simulink model "ComputedTorqueControl_20220607"  (R2020a)
settings: Solver=VariableStepAuto  StartTime=0.0  StopTime=12  FixedStep=0.01  RelTol=1e-3
undefined symbols (not defined in the file or in its folder): X, Y, Z
libraries: sm_lib x197, nesl_utility x84, sm_cable_robot_lib x44, simulink x1
(part 8 of 8)

== system ComputedTorqueControl_20220607/4-DOF CDPR/Frame2/Column 4/Lower Motor Assembly/Motor ==
  Double Bracket : Subsystem  AncestorBlock=sm_cable_robot_lib/Double Bracket  mask(Double Bracket){height=0.05, width=0.02, thickness=0.002, offset=0.13, holeOffset=0.04, holeRadius=0.005, rho=7800, color=[0.5 0.5 0.5]}
      mask prompts: height "Height (m)"; width "Width (m)"; thickness "Thickness (m)"; offset "Offset (m)"; holeOffset "Hole Offset (m)"; holeRadius "Hole Radius (m)"; rho "Density (kg/m^3)"; color "Color [r g b]"
      mask help:
      | This block models a double bracket element.
      |
      | Port B corresponds to the midpoint between the base faces of the two elements. Port H corresponds to the midpoint between the two holes.
      mask DialogControl Tab1 Prompt: Dimensions
      mask DialogControl Tab2 Prompt: Material Properties
      mask Display: image(fullfile(matlabroot,'toolbox','physmod','sm','smdemos','cable_robot','images','sm_cable_robot_double_bracket.png'));
  Flange : sm_lib/Body Elements/Cylindrical Solid  GraphicAmbientColor=[0.15 0.15 0.15 1.0]  BasedOnType=Density  CenterOfMass=[0 0 0]  CenterOfMassUnits=m  GraphicDiffuseColor=flangeColor  CylinderLength=flangeThickness  CylinderLengthUnits=m  CylinderRadius=flangeRadius  CylinderRadiusUnits=m  Density=housingRho  DensityUnits=kg/m^3  DoExposeReferenceFrame=off  GraphicEmissiveColor=[0.0 0.0 0.0 1.0]  ExportEntireGeometry=off  SerializedFrames=<Frames><Frame><Id>Frame1</Id><Value><Name>B</Name><Origin><Source>GeometricFeature</Source><FeatureName>bottom surface</FeatureName></Origin><PrimaryAxis><DefinedDirection>+Z</DefinedDirection><Source>ReferenceFrame</Source><SourceDirection>+Z</SourceDirection><FeatureName></FeatureName></PrimaryAxis><SecondaryAxis><DefinedDirection>+X</DefinedDirection><Source>ReferenceFrame</Source><SourceDirection>+X</SourceDirection><FeatureName></FeatureName></SecondaryAxis></Value></Frame></Frames>  MarkerShape=Sphere  MarkerSize=10  GraphicType=FromGeometry  InertiaType=CalculateFromGeometry  Mass=1  MassUnits=kg  MomentsOfInertia=[1 1 1]  MomentsOfInertiaUnits=kg*m^2  GraphicOpacity=1.0  ProductsOfInertia=[0 0 0]  ProductsOfInertiaUnits=kg*m^2  GraphicShininess=75  GraphicSpecularColor=[0.5 0.5 0.5 1.0]  GraphicVisPropType=SimpleVisualProperties
  Housing : sm_lib/Body Elements/Brick Solid  GraphicAmbientColor=[0.15 0.15 0.15 1.0]  BasedOnType=Density  BrickDimensions=[width height depth]  BrickDimensionUnits=m  CenterOfMass=[0 0 0]  CenterOfMassUnits=m  GraphicDiffuseColor=housingColor  Density=housingRho  DensityUnits=kg/m^3  DoExposeReferenceFrame=off  GraphicEmissiveColor=[0.0 0.0 0.0 1.0]  ExportEntireGeometry=off  SerializedFrames=<Frames><Frame><Id>Frame2</Id><Value><Name>B</Name><Origin><Source>GeometricFeature</Source><FeatureName>-y surface</FeatureName></Origin><PrimaryAxis><DefinedDirection>+Z</DefinedDirection><Source>ReferenceFrame</Source><SourceDirection>+Z</SourceDirection><FeatureName></FeatureName></PrimaryAxis><SecondaryAxis><DefinedDirection>+X</DefinedDirection><Source>ReferenceFrame</Source><SourceDirection>+X</SourceDirection><FeatureName></FeatureName></SecondaryAxis></Value></Frame><Frame><Id>Frame3</Id><Value><Name>F</Name><Origin><Source>GeometricFeature</Source><FeatureName>+z surface</FeatureName></Origin><PrimaryAxis><DefinedDirection>+Z</DefinedDirection><Source>ReferenceFrame</Source><SourceDirection>+Z</SourceDirection><FeatureName></FeatureName></PrimaryAxis><SecondaryAxis><DefinedDirection>+X</DefinedDirection><Source>ReferenceFrame</Source><SourceDirection>+X</SourceDirection><FeatureName></FeatureName></SecondaryAxis></Value></Frame></Frames>  MarkerShape=Sphere  MarkerSize=10  GraphicType=FromGeometry  InertiaType=CalculateFromGeometry  Mass=1  MassUnits=kg  MomentsOfInertia=[1 1 1]  MomentsOfInertiaUnits=kg*m^2  GraphicOpacity=1.0  ProductsOfInertia=[0 0 0]  ProductsOfInertiaUnits=kg*m^2  GraphicShininess=75  GraphicSpecularColor=[0.5 0.5 0.5 1.0]  GraphicVisPropType=SimpleVisualProperties
  Motor Revolute : sm_lib/Joints/Revolute Joint  JointMode=Normal  SenseConstraintForce=off  SenseConstraintForceX=off  SenseConstraintForceY=off  SenseConstraintForceZ=off  SenseConstraintTorque=off  SenseConstraintTorqueX=off  SenseConstraintTorqueY=off  SenseConstraintTorqueZ=off  SenseTotalForce=off  SenseTotalForceX=off  SenseTotalForceY=off  SenseTotalForceZ=off  SenseTotalTorque=off  SenseTotalTorqueX=off  SenseTotalTorqueY=off  SenseTotalTorqueZ=off  CompositeWrenchDir=FollowerOnBase  CompositeWrenchFrame=BaseFrame  EquilibriumPosition=0  EquilibriumPositionUnits=deg  SpringStiffness=0  SpringStiffnessUnits=N*m/deg  DampingCoefficient=0.01  DampingCoefficientUnits=N*m/(deg/s)  TorqueActuationMode=InputTorque  MotionActuationMode=ComputedMotion  SensePosition=on  SenseVelocity=on  SenseAcceleration=on  SenseTorqueForce=on  SenseLowerLimitTorqueForce=off  SenseUpperLimitTorqueForce=off  LowerLimitSpecify=off  LowerLimitBound=-90  LowerLimitBoundUnits=deg  LowerLimitStiffness=1e4  LowerLimitStiffnessUnits=N*m/deg  LowerLimitDamping=10  LowerLimitDampingUnits=N*m/(deg/s)  LowerLimitTransitionRegionWidth=0.1  LowerLimitTransitionRegionWidthUnits=deg  UpperLimitSpecify=off  UpperLimitBound=90  UpperLimitBoundUnits=deg  UpperLimitStiffness=1e4  UpperLimitStiffnessUnits=N*m/deg  UpperLimitDamping=10  UpperLimitDampingUnits=N*m/(deg/s)  UpperLimitTransitionRegionWidth=0.1  UpperLimitTransitionRegionWidthUnits=deg  PositionTargetSpecify=off  PositionTargetPriority=High  PositionTargetValue=0  PositionTargetValueUnits=deg  VelocityTargetSpecify=off  VelocityTargetPriority=High  VelocityTargetValue=0  VelocityTargetValueUnits=deg/s
  PS-Simulink Converter{1..4} (4 alike) : nesl_utility/PS-Simulink Converter  PhysicalDomain=network_engine_domain  SubClassName=ps_output  LeftPortType=input  RightPortType=output  PseudoPeriodic=off  Frequencies=[]  Unit=inherit  AffineConversion=off
  Rigid Transform : sm_lib/Frames and Transforms/Rigid Transform  TranslationMethod=Cartesian  TranslationStandardOffset=0  TranslationLengthUnit=m  TranslationStandardAxis=+Z  TranslationCartesianOffset=[0 -0.04 0.075]  TranslationROffset=0  TranslationROffsetUnits=m  TranslationZOffset=0  TranslationZOffsetUnits=m  TranslationThetaOffset=0  TranslationThetaOffsetUnits=deg  RotationMethod=RotationSequence  RotationAngleUnits=deg  RotationStandardAxis=+X  RotationAngle=90  RotationArbitraryAxis=[0 0 1]  FollAlignAxisA=+X  BaseAlignAxisA=+Y  FollAlignAxisB=+Y  BaseAlignAxisB=+Z  RotationSequenceAxes=FollowerAxes  RotationSequence=XYZ  RotationSequenceAngles=[-90 0 0]  RotationSequenceAnglesUnits=deg  RotationMatrix=[1 0 0; 0 1 0; 0 0 1]
  Shaft : sm_lib/Body Elements/Cylindrical Solid  GraphicAmbientColor=[0.15 0.15 0.15 1.0]  BasedOnType=Density  CenterOfMass=[0 0 0.075]  CenterOfMassUnits=m  GraphicDiffuseColor=shaftColor  CylinderLength=shaftLength  CylinderLengthUnits=m  CylinderRadius=shaftRadius  CylinderRadiusUnits=m  Density=shaftRho  DensityUnits=kg/m^3  DoExposeReferenceFrame=on  GraphicEmissiveColor=[0.0 0.0 0.0 1.0]  ExportEntireGeometry=off  SerializedFrames=<Frames><Frame><Id>Frame1</Id><Value><Name>B</Name><Origin><Source>GeometricFeature</Source><FeatureName>bottom surface</FeatureName></Origin><PrimaryAxis><DefinedDirection>+Z</DefinedDirection><Source>ReferenceFrame</Source><SourceDirection>+Z</SourceDirection><FeatureName></FeatureName></PrimaryAxis><SecondaryAxis><DefinedDirection>+X</DefinedDirection><Source>ReferenceFrame</Source><SourceDirection>+X</SourceDirection><FeatureName></FeatureName></SecondaryAxis></Value></Frame></Frames>  MarkerShape=Sphere  MarkerSize=10  GraphicType=FromGeometry  InertiaType=Custom  Mass=0.09189  MassUnits=kg  MomentsOfInertia=[0 0 1.149e-6]  MomentsOfInertiaUnits=kg*m^2  GraphicOpacity=1.0  ProductsOfInertia=[0 0 0]  ProductsOfInertiaUnits=kg*m^2  GraphicShininess=75  GraphicSpecularColor=[0.5 0.5 0.5 1.0]  GraphicVisPropType=SimpleVisualProperties
  Simulink-PS Converter : nesl_utility/Simulink-PS Converter  PhysicalDomain=network_engine_domain  SubClassName=ps_input  LeftPortType=input  RightPortType=output  PseudoPeriodic=off  Frequencies=[]  NoiseDistribution=none  NoiseParameters=[]  Unit=N*m  AffineConversion=off  FilteringAndDerivatives=filter  SimscapeFilterOrder=2  InputFilterTimeConstant=0.001  UdotUserProvided=0
  To Workspace1 : ToWorkspace  VariableName=qD  SaveFormat=Structure With Time  SampleTime=-1
  To Workspace2 : ToWorkspace  VariableName=dqD  SaveFormat=Structure With Time  SampleTime=-1
  To Workspace3 : ToWorkspace  VariableName=ddqD  SaveFormat=Structure With Time  SampleTime=-1
  To Workspace4 : ToWorkspace  VariableName=Dtrq  SaveFormat=Structure With Time  SampleTime=-1
  B : PMIOPort  Side=Left
  S : PMIOPort  Port=2  Side=Right
  tag scope: Dtrq=global, ddqD=global, dqD=global, qD=global
  wires:
  [DInTorque] -> Simulink-PS Converter/1
  PS-Simulink Converter3/1 -> To Workspace3/1, [ddqD]
  PS-Simulink Converter2/1 -> To Workspace2/1, [dqD]
  PS-Simulink Converter4/1 -> To Workspace4/1, [Dtrq]
  PS-Simulink Converter1/1 -> To Workspace1/1, [qD]
  connections:
  Housing/LConn1 -- B/RConn1
  S/RConn1 -- Shaft/RConn1
  Shaft/LConn1 -- Motor Revolute/RConn1
  Flange/LConn1 -- Housing/RConn1 -- Rigid Transform/LConn1 -- Motor Revolute/LConn1
  Rigid Transform/RConn1 -- Double Bracket/LConn1
  Simulink-PS Converter/RConn1 -- Motor Revolute/LConn2
  PS-Simulink Converter3/LConn1 -- Motor Revolute/RConn4
  PS-Simulink Converter1/LConn1 -- Motor Revolute/RConn2
  PS-Simulink Converter4/LConn1 -- Motor Revolute/RConn5
  PS-Simulink Converter2/LConn1 -- Motor Revolute/RConn3

== system ComputedTorqueControl_20220607/4-DOF CDPR/Frame2/Column 4/Lower Motor Assembly/Pulley and Bracket Assembly ==
  Pulley : sm_cable_robot_lib/Pulley  radius=0.02  thickness=0.12  holeRadius=0.005  grooveDepth=0.004  grooveWidth=0.1  grooveAngle=25  rho=7800  color=[0.7 0.7 0.7]  markerColor=[0.3 0.3 0.3]
      link override Pulley: CenterOfMass=[0 0 0.1]  InertiaType=Custom  Mass=1.8378  MomentsOfInertia=[0 0 3.905e-4]
      settings: SourceProductBaseCode=MS
  Rigid Transform1 : sm_lib/Frames and Transforms/Rigid Transform  TranslationMethod=None  TranslationStandardOffset=0  TranslationLengthUnit=m  TranslationStandardAxis=+Z  TranslationCartesianOffset=[0 0 0]  TranslationROffset=0  TranslationROffsetUnits=m  TranslationZOffset=0  TranslationZOffsetUnits=m  TranslationThetaOffset=0  TranslationThetaOffsetUnits=deg  RotationMethod=None  RotationAngleUnits=deg  RotationStandardAxis=+X  RotationAngle=90  RotationArbitraryAxis=[0 0 1]  FollAlignAxisA=+X  BaseAlignAxisA=+Y  FollAlignAxisB=+Y  BaseAlignAxisB=+Z  RotationSequenceAxes=FollowerAxes  RotationSequence=XYZ  RotationSequenceAngles=[-90 0 0]  RotationSequenceAnglesUnits=deg  RotationMatrix=[1 0 0; 0 1 0; 0 0 1]
  B : PMIOPort  Side=Left
  connections:
  Rigid Transform1/RConn1 -- Pulley/LConn1
  B/RConn1 -- Rigid Transform1/LConn1

== system ComputedTorqueControl_20220607/4-DOF CDPR/Frame2/Column 1/Lower Motor Assembly/Motor/Double Bracket ==
  Base Center Frame : sm_lib/Frames and Transforms/Reference Frame
  Left Bracket : sm_cable_robot_lib/Bracket  height=height  width=width  thickness=thickness  holeOffset=holeOffset  holeRadius=holeRadius  rho=rho  color=color
      settings: SourceProductBaseCode=MS
  Left Bracket xForm : sm_lib/Frames and Transforms/Rigid Transform  TranslationMethod=StandardAxis  TranslationStandardOffset=0.5*offset  TranslationLengthUnit=m  TranslationStandardAxis=-Y  TranslationCartesianOffset=[0 0 0]  TranslationROffset=0  TranslationROffsetUnits=m  TranslationZOffset=0  TranslationZOffsetUnits=m  TranslationThetaOffset=0  TranslationThetaOffsetUnits=deg  RotationMethod=AlignedAxes  RotationAngleUnits=deg  RotationStandardAxis=+X  RotationAngle=90  RotationArbitraryAxis=[0 0 1]  FollAlignAxisA=+X  BaseAlignAxisA=+X  FollAlignAxisB=+Y  BaseAlignAxisB=+Z  RotationSequenceAxes=FollowerAxes  RotationSequence=XYX  RotationSequenceAngles=[0 0 0]  RotationSequenceAnglesUnits=deg  RotationMatrix=[1 0 0; 0 1 0; 0 0 1]
  Right Bracket : sm_cable_robot_lib/Bracket  height=height  width=width  thickness=thickness  holeOffset=holeOffset  holeRadius=holeRadius  rho=rho  color=color
      settings: SourceProductBaseCode=MS
  Right Bracket xForm : sm_lib/Frames and Transforms/Rigid Transform  TranslationMethod=StandardAxis  TranslationStandardOffset=0.5*offset  TranslationLengthUnit=m  TranslationStandardAxis=+Y  TranslationCartesianOffset=[0 0 0]  TranslationROffset=0  TranslationROffsetUnits=m  TranslationZOffset=0  TranslationZOffsetUnits=m  TranslationThetaOffset=0  TranslationThetaOffsetUnits=deg  RotationMethod=AlignedAxes  RotationAngleUnits=deg  RotationStandardAxis=+X  RotationAngle=90  RotationArbitraryAxis=[0 0 1]  FollAlignAxisA=+X  BaseAlignAxisA=+X  FollAlignAxisB=+Y  BaseAlignAxisB=+Z  RotationSequenceAxes=FollowerAxes  RotationSequence=XYX  RotationSequenceAngles=[0 0 0]  RotationSequenceAnglesUnits=deg  RotationMatrix=[1 0 0; 0 1 0; 0 0 1]
  B : PMIOPort  Side=Left
  connections:
  B/RConn1 -- Base Center Frame/RConn1 -- Right Bracket xForm/LConn1 -- Left Bracket xForm/LConn1
  Right Bracket/LConn1 -- Right Bracket xForm/RConn1
  Left Bracket/LConn1 -- Left Bracket xForm/RConn1

== system ComputedTorqueControl_20220607/4-DOF CDPR/Frame2/Column 2/Lower Motor Assembly1/Motor/Double Bracket ==
  Base Center Frame : sm_lib/Frames and Transforms/Reference Frame
  Left Bracket : sm_cable_robot_lib/Bracket  height=height  width=width  thickness=thickness  holeOffset=holeOffset  holeRadius=holeRadius  rho=rho  color=color
      settings: SourceProductBaseCode=MS
  Left Bracket xForm : sm_lib/Frames and Transforms/Rigid Transform  TranslationMethod=StandardAxis  TranslationStandardOffset=0.5*offset  TranslationLengthUnit=m  TranslationStandardAxis=-Y  TranslationCartesianOffset=[0 0 0]  TranslationROffset=0  TranslationROffsetUnits=m  TranslationZOffset=0  TranslationZOffsetUnits=m  TranslationThetaOffset=0  TranslationThetaOffsetUnits=deg  RotationMethod=AlignedAxes  RotationAngleUnits=deg  RotationStandardAxis=+X  RotationAngle=90  RotationArbitraryAxis=[0 0 1]  FollAlignAxisA=+X  BaseAlignAxisA=+X  FollAlignAxisB=+Y  BaseAlignAxisB=+Z  RotationSequenceAxes=FollowerAxes  RotationSequence=XYX  RotationSequenceAngles=[0 0 0]  RotationSequenceAnglesUnits=deg  RotationMatrix=[1 0 0; 0 1 0; 0 0 1]
  Right Bracket : sm_cable_robot_lib/Bracket  height=height  width=width  thickness=thickness  holeOffset=holeOffset  holeRadius=holeRadius  rho=rho  color=color
      settings: SourceProductBaseCode=MS
  Right Bracket xForm : sm_lib/Frames and Transforms/Rigid Transform  TranslationMethod=StandardAxis  TranslationStandardOffset=0.5*offset  TranslationLengthUnit=m  TranslationStandardAxis=+Y  TranslationCartesianOffset=[0 0 0]  TranslationROffset=0  TranslationROffsetUnits=m  TranslationZOffset=0  TranslationZOffsetUnits=m  TranslationThetaOffset=0  TranslationThetaOffsetUnits=deg  RotationMethod=AlignedAxes  RotationAngleUnits=deg  RotationStandardAxis=+X  RotationAngle=90  RotationArbitraryAxis=[0 0 1]  FollAlignAxisA=+X  BaseAlignAxisA=+X  FollAlignAxisB=+Y  BaseAlignAxisB=+Z  RotationSequenceAxes=FollowerAxes  RotationSequence=XYX  RotationSequenceAngles=[0 0 0]  RotationSequenceAnglesUnits=deg  RotationMatrix=[1 0 0; 0 1 0; 0 0 1]
  B : PMIOPort  Side=Left
  connections:
  B/RConn1 -- Base Center Frame/RConn1 -- Right Bracket xForm/LConn1 -- Left Bracket xForm/LConn1
  Right Bracket/LConn1 -- Right Bracket xForm/RConn1
  Left Bracket/LConn1 -- Left Bracket xForm/RConn1

== system ComputedTorqueControl_20220607/4-DOF CDPR/Frame2/Column 3/Lower Motor Assembly/Motor/Double Bracket ==
  Base Center Frame : sm_lib/Frames and Transforms/Reference Frame
  Left Bracket : sm_cable_robot_lib/Bracket  height=height  width=width  thickness=thickness  holeOffset=holeOffset  holeRadius=holeRadius  rho=rho  color=color
      settings: SourceProductBaseCode=MS
  Left Bracket xForm : sm_lib/Frames and Transforms/Rigid Transform  TranslationMethod=StandardAxis  TranslationStandardOffset=0.5*offset  TranslationLengthUnit=m  TranslationStandardAxis=-Y  TranslationCartesianOffset=[0 0 0]  TranslationROffset=0  TranslationROffsetUnits=m  TranslationZOffset=0  TranslationZOffsetUnits=m  TranslationThetaOffset=0  TranslationThetaOffsetUnits=deg  RotationMethod=AlignedAxes  RotationAngleUnits=deg  RotationStandardAxis=+X  RotationAngle=90  RotationArbitraryAxis=[0 0 1]  FollAlignAxisA=+X  BaseAlignAxisA=+X  FollAlignAxisB=+Y  BaseAlignAxisB=+Z  RotationSequenceAxes=FollowerAxes  RotationSequence=XYX  RotationSequenceAngles=[0 0 0]  RotationSequenceAnglesUnits=deg  RotationMatrix=[1 0 0; 0 1 0; 0 0 1]
  Right Bracket : sm_cable_robot_lib/Bracket  height=height  width=width  thickness=thickness  holeOffset=holeOffset  holeRadius=holeRadius  rho=rho  color=color
      settings: SourceProductBaseCode=MS
  Right Bracket xForm : sm_lib/Frames and Transforms/Rigid Transform  TranslationMethod=StandardAxis  TranslationStandardOffset=0.5*offset  TranslationLengthUnit=m  TranslationStandardAxis=+Y  TranslationCartesianOffset=[0 0 0]  TranslationROffset=0  TranslationROffsetUnits=m  TranslationZOffset=0  TranslationZOffsetUnits=m  TranslationThetaOffset=0  TranslationThetaOffsetUnits=deg  RotationMethod=AlignedAxes  RotationAngleUnits=deg  RotationStandardAxis=+X  RotationAngle=90  RotationArbitraryAxis=[0 0 1]  FollAlignAxisA=+X  BaseAlignAxisA=+X  FollAlignAxisB=+Y  BaseAlignAxisB=+Z  RotationSequenceAxes=FollowerAxes  RotationSequence=XYX  RotationSequenceAngles=[0 0 0]  RotationSequenceAnglesUnits=deg  RotationMatrix=[1 0 0; 0 1 0; 0 0 1]
  B : PMIOPort  Side=Left
  connections:
  B/RConn1 -- Base Center Frame/RConn1 -- Right Bracket xForm/LConn1 -- Left Bracket xForm/LConn1
  Right Bracket/LConn1 -- Right Bracket xForm/RConn1
  Left Bracket/LConn1 -- Left Bracket xForm/RConn1

== system ComputedTorqueControl_20220607/4-DOF CDPR/Frame2/Column 4/Lower Motor Assembly/Motor/Double Bracket ==
  Base Center Frame : sm_lib/Frames and Transforms/Reference Frame
  Left Bracket : sm_cable_robot_lib/Bracket  height=height  width=width  thickness=thickness  holeOffset=holeOffset  holeRadius=holeRadius  rho=rho  color=color
      settings: SourceProductBaseCode=MS
  Left Bracket xForm : sm_lib/Frames and Transforms/Rigid Transform  TranslationMethod=StandardAxis  TranslationStandardOffset=0.5*offset  TranslationLengthUnit=m  TranslationStandardAxis=-Y  TranslationCartesianOffset=[0 0 0]  TranslationROffset=0  TranslationROffsetUnits=m  TranslationZOffset=0  TranslationZOffsetUnits=m  TranslationThetaOffset=0  TranslationThetaOffsetUnits=deg  RotationMethod=AlignedAxes  RotationAngleUnits=deg  RotationStandardAxis=+X  RotationAngle=90  RotationArbitraryAxis=[0 0 1]  FollAlignAxisA=+X  BaseAlignAxisA=+X  FollAlignAxisB=+Y  BaseAlignAxisB=+Z  RotationSequenceAxes=FollowerAxes  RotationSequence=XYX  RotationSequenceAngles=[0 0 0]  RotationSequenceAnglesUnits=deg  RotationMatrix=[1 0 0; 0 1 0; 0 0 1]
  Right Bracket : sm_cable_robot_lib/Bracket  height=height  width=width  thickness=thickness  holeOffset=holeOffset  holeRadius=holeRadius  rho=rho  color=color
      settings: SourceProductBaseCode=MS
  Right Bracket xForm : sm_lib/Frames and Transforms/Rigid Transform  TranslationMethod=StandardAxis  TranslationStandardOffset=0.5*offset  TranslationLengthUnit=m  TranslationStandardAxis=+Y  TranslationCartesianOffset=[0 0 0]  TranslationROffset=0  TranslationROffsetUnits=m  TranslationZOffset=0  TranslationZOffsetUnits=m  TranslationThetaOffset=0  TranslationThetaOffsetUnits=deg  RotationMethod=AlignedAxes  RotationAngleUnits=deg  RotationStandardAxis=+X  RotationAngle=90  RotationArbitraryAxis=[0 0 1]  FollAlignAxisA=+X  BaseAlignAxisA=+X  FollAlignAxisB=+Y  BaseAlignAxisB=+Z  RotationSequenceAxes=FollowerAxes  RotationSequence=XYX  RotationSequenceAngles=[0 0 0]  RotationSequenceAnglesUnits=deg  RotationMatrix=[1 0 0; 0 1 0; 0 0 1]
  B : PMIOPort  Side=Left
  connections:
  B/RConn1 -- Base Center Frame/RConn1 -- Right Bracket xForm/LConn1 -- Left Bracket xForm/LConn1
  Right Bracket/LConn1 -- Right Bracket xForm/RConn1
  Left Bracket/LConn1 -- Left Bracket xForm/RConn1

== matlab function ComputedTorqueControl_20220607/Reference Trajectory Generator/Subsystem/MATLAB Function2 ==
  data: t input; Adq output; Bdq output; Cdq output; Ddq output
function [Adq,Bdq,Cdq,Ddq] = fcn(t)

 Adq=(-t+2).*(0<=t&&t<=4)+(t-8).*(4<=t&&t<=12);
 Bdq=(-t+4).*(0<=t&&t<=8)+(t-10).*(8<=t&&t<=12);
 Cdq=(t-2).*(0<=t&&t<=4)+(-t+8).*(4<=t&&t<=12);
 Ddq=(t-4).*(0<=t&&t<=8)+(-t+10).*(8<=t&&t<=12);
end

== matlab function ComputedTorqueControl_20220607/Reference Trajectory Generator/Subsystem/MATLAB Function1 ==
  data: t input; Aq output; Bq output; Cq output; Dq output
function [Aq,Bq,Cq,Dq] = fcn(t)

  Aq=(-0.5*(t-2)^2+2).*(0<=t&&t<4)+(0.5*(t-8)^2-8).*(4<=t&&t<12);
  Bq=(-0.5*(t-4)^2+8).*(0<=t&&t<8)+(0.5*(t-10)^2-2).*(8<t&&t<12);
  Cq=(0.5*(t-2)^2-2).*(0<t&&t<=4)+(-0.5*(t-8)^2+8).* (4<t&&t<12);
  Dq=(0.5*(t-4)^2-8).*(0<t&&t<=8)+(-0.5*(t-10)^2+2).* (8<t&&t<12);
 
end

== matlab function ComputedTorqueControl_20220607/Reference Trajectory Generator/Subsystem/MATLAB Function3 ==
  data: t input; Addq output; Bddq output; Cddq output; Dddq output
function [Addq,Bddq,Cddq,Dddq] = fcn(t)

Addq=-1.801*t+11.63;
Bddq=-4.122*t+38.26;
Cddq=1.801*t-11.63;
Dddq=4.122*t-38.26;

end

== matlab function ComputedTorqueControl_20220607/Reference Trajectory Generator/Subsystem/MATLAB Function4 ==
  data: t input; Aq output; Bq output; Cq output; Dq output
function [Aq,Bq,Cq,Dq] = fcn(t)

  Aq=3.994*sin(0.1796*t-2.995) + 4.244*sin(0.5746*t+0.1555);
  Bq=19.81*sin(0.002025*t+2.993) + 5.099*sin(0.5257*t-0.6065);
  Cq=18.34*sin(0.002452*t+0.1331) + 5.084*sin(0.5268*t-2.588);
  Dq=4.038*sin(0.1823*t+0.1823) + 4.202*sin(0.5769*t+2.34);
 
end

== matlab function ComputedTorqueControl_20220607/Reference Trajectory Generator/Subsystem/MATLAB Function ==
  data: t input; Atau output; Btau output; Ctau output; Dtau output
function [Atau,Btau,Ctau,Dtau] = fcn(t)

Atau= 2.721*sin(0.525*t+2.124);
Btau=2.724*sin(0.5233*t+0.9912);
Ctau=2.727*sin(0.5209*t-0.9968);
Dtau=2.722*sin(0.5277*t-2.18);

end

== matlab function ComputedTorqueControl_20220607/Tension Force ==
  data: q input; f output; al input; be input; ga input
function f = Tension_Force(q,al,be,ga)

% %定义的电机转角q;q=[q1;q2;q3;q4];
q1=q(1);q2=q(2);q3=q(3);q4=q(4);

 % %定义的零位置的悬索（未形变）长度L00：
L0=[2.0992    1.9280    1.5225    1.6912    2.0992    1.9280    1.5225    1.6912]';
l01=L0(1,1);l02=L0(2,1);l03=L0(3,1);l04=L0(4,1);
l05=L0(5,1);l06=L0(6,1);l07=L0(7,1);l08=L0(8,1);
 
% %⑥悬索未形变的长度Lo。初始点位置为[0；0；1.1；0；0；0]。
% l0=1.7305*a0;
r0=0.02;
% m0=5.826*10^(-4);
lo1=l01+r0*q1;lo2=l02+r0*q2;lo3=l03+r0*q3;lo4=l04+r0*q4;
lo5=l05+r0*q1;lo6=l06+r0*q2;lo7=l07+r0*q3;lo8=l08+r0*q4;

%执行器位置参数
x=1.1;y=1.5;z=0.75;
%外框架尺寸设定
A=2.2;B=3.0;C=1.5;
a=0.2;b=0.05;h=0.1;


P=[x;y;z];
% R=[cos(ga),-sin(ga),0;sin(ga),cos(ga),0;0,0,1];
R=[cos(ga)*cos(be),  cos(ga)*sin(be)*sin(al)-sin(ga)*cos(al),  cos(ga)*sin(be)*cos(al)+sin(ga)*sin(al);  
   sin(ga)*cos(be),  sin(ga)*sin(be)*sin(al)+cos(ga)*cos(al),  sin(ga)*sin(be)*cos(al)-cos(ga)*sin(al);   
          -sin(be),                          cos(be)*sin(al),                        cos(be)*cos(al)   ];       
% %全局坐标原点O位于外框架接地平面中心。局部坐标系原点建立在末端执行器中心。
B1=[A/2;B/2;   C];B2=[-A/2;B/2;   C];B3=[-A/2;-B/2;   C];B4=[A/2;-B/2;  C];
B5=[A/2;B/2; C-h];B6=[-A/2;B/2; C-h];B7=[-A/2;-B/2; C-h];B8=[A/2;-B/2; C-h];
p1=[a/2;b/2; h/2];p2=[-a/2;b/2; h/2];p3=[-a/2;-b/2; h/2];p4=[a/2;-b/2; h/2];
p5=[a/2;b/2;-h/2];p6=[-a/2;b/2;-h/2];p7=[-a/2;-b/2;-h/2];p8=[a/2;-b/2;-h/2];
% %悬索矢量。
L1=P+R*p1-B1;L2=P+R*p2-B2;L3=P+R*p3-B3;L4=P+R*p4-B4;L5=P+R*p5-B5;L6=P+R*p6-B6;L7=P+R*p7-B7;L8=P+R*p8-B8;
le1=norm(L1);le2=norm(L2);le3=norm(L3);le4=norm(L4);le5=norm(L5);le6=norm(L6);le7=norm(L7);le8=norm(L8);

% %⑧悬索形变量：Loe1，Loe2,...,Loe8;
Loe1=[lo1-le1;lo2-le2;lo3-le3;lo4-le4;];
Loe2=[lo5-le5;lo6-le6;lo7-le7;lo8-le8;];
Loe=Loe1+Loe2;
LoeA=Loe(1);LoeB=Loe(2);LoeC=Loe(3);LoeD=Loe(4);

% % 绳索横截面积以及弹性模量
%E=43.9*10^6;SA=3.14*10^(-6) ;K0=E*SA;
K0=100;

% %刚度矩阵K(Lo)
%K =diag([K0/lo1,K0/lo2,K0/lo3,K0/lo4,K0/lo5,K0/lo6,K0/lo7,K0/lo8]);
K1=K0/lo1;K2=K0/lo2;K3=K0/lo3;K4=K0/lo4;


% %含弹性形变的拉力求解
f1 = K1.* LoeA;f2 = K2.* LoeB;f3 = K3.* LoeC;f4 = K4.* LoeD;
f = [f1;f2;f3;f4;];

end
